simulink model "PruebaLEDs"  (R2023b)
settings: Solver=FixedStepAuto  StartTime=0.0  StopTime=inf  RelTol=1e-3
libraries: arduinolib x3
settings Model: Creator=Usuario_UMA  LastModifiedBy=Diego
settings OptimizationCC: DefaultParameterBehavior=Inlined  EnhancedBackFolding=on  PassReuseOutputArgsAs=Individual arguments  ZeroExternalMemoryAtStartup=off  ZeroInternalMemoryAtStartup=off  MaxStackSize=64  OptimizeBlockOrder=speed  DifferentSizesBufferReuse=on  OptimizationCustomize=off  EfficientTunableParamExpr=on
settings DebuggingCC: ParameterTunabilityLossMsg=error
settings HardwareCC: ProdBitPerInt=16  ProdBitPerPointer=16  ProdBitPerSizeT=16  ProdBitPerPtrDiffT=16  ProdLargestAtomicFloat=None  ProdWordSize=8  ProdHWDeviceType=Atmel->AVR
settings SFSimCC: MATLABDynamicMemAlloc=off
settings RTWCC: Description=Embedded Coder  SystemTargetFile=ert.tlc  TemplateMakefile=ert_default_tmf  Toolchain=Arduino AVR  BuildConfiguration=Faster Runs
settings CodeAppCC: ForceParamTrailComments=on  IgnoreCustomStorageClasses=off  OperatorAnnotations=on  SimulinkDataObjDesc=on  SFDataObjDesc=on  InsertBlockDesc=on
settings ERTTargetCC: SupportContinuousTime=on  ExtModeTransport=3  ExtModeStaticAlloc=on  ExtModeStaticAllocSize=2048  ExtModeMexFile=ext_xcp  ExtModeIntrfLevel=Level2 - Open  ERTCustomFileTemplate=example_file_process.tlc

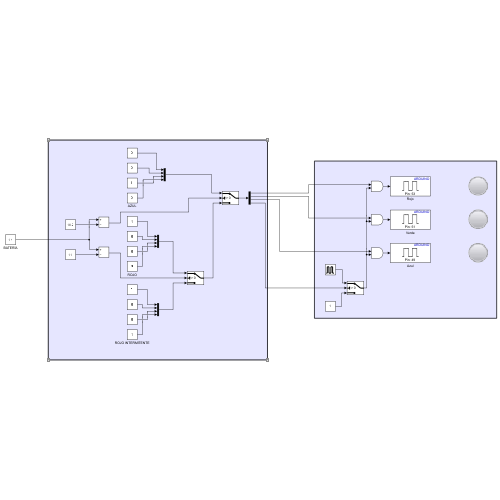
[thumbnail: Simulink's stored preview of the top-level diagram]
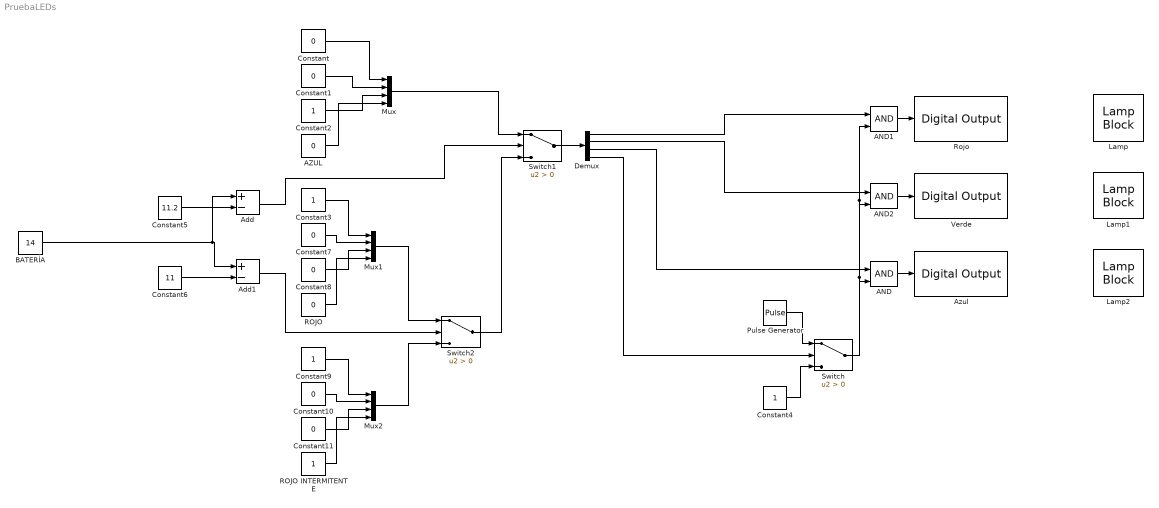
== system PruebaLEDs ==
  AND : Logic  IconShape=distinctive  AllPortsSameDT=off  OutDataTypeStr=boolean
  AND1 : Logic  IconShape=distinctive  AllPortsSameDT=off  OutDataTypeStr=boolean
  AND2 : Logic  IconShape=distinctive  AllPortsSameDT=off  OutDataTypeStr=boolean
  AZUL : Constant  Value=0
  Add : Sum  Inputs=+-
  Add1 : Sum  Inputs=+-
  Azul : arduinolib/Digital Output  pinNumber=49  Direction=output  blockPlatform=arduino
  BATERÍA : Constant  Value=14
  Constant{,1,7..8,10..11} (6 alike) : Constant  Value=0
  Constant{2..4,9} (4 alike) : Constant
  Constant5 : Constant  Value=11.2
  Constant6 : Constant  Value=11
  Demux : Demux
  Lamp : LampBlock  LabelPosition=Hide
  Lamp1 : LampBlock  LabelPosition=Hide
  Lamp2 : LampBlock  LabelPosition=Hide
  Mux : Mux
  Mux1 : Mux
  Mux2 : Mux
  Pulse Generator : DiscretePulseGenerator  PulseType=Time based  Period=1  PulseWidth=50
  ROJO : Constant  Value=0
  ROJO INTERMITENTE : Constant
  Rojo : arduinolib/Digital Output  pinNumber=53  Direction=output  blockPlatform=arduino
  Switch : Switch  Criteria=u2 > Threshold  SaturateOnIntegerOverflow=off  InputSameDT=off
  Switch1 : Switch  Criteria=u2 > Threshold  SaturateOnIntegerOverflow=off  InputSameDT=off
  Switch2 : Switch  Criteria=u2 > Threshold  SaturateOnIntegerOverflow=off  InputSameDT=off
  Verde : arduinolib/Digital Output  pinNumber=51  Direction=output  blockPlatform=arduino
  wires:
  AND/1 -> Azul/1
  Switch/1 -> AND2/2, AND1/2, AND/2
  Pulse Generator/1 -> Switch/1
  Constant4/1 -> Switch/3
  AND1/1 -> Rojo/1
  AND2/1 -> Verde/1
  Constant/1 -> Mux/1
  Constant1/1 -> Mux/2
  Constant2/1 -> Mux/3
  AZUL/1 -> Mux/4
  Constant3/1 -> Mux1/1
  Constant7/1 -> Mux1/2
  Constant8/1 -> Mux1/3
  ROJO/1 -> Mux1/4
  Constant9/1 -> Mux2/1
  Constant10/1 -> Mux2/2
  Constant11/1 -> Mux2/3
  ROJO INTERMITENTE/1 -> Mux2/4
  BATERÍA/1 -> Add/1, Add1/1
  Constant5/1 -> Add/2
  Constant6/1 -> Add1/2
  Add/1 -> Switch1/2
  Mux/1 -> Switch1/1
  Mux1/1 -> Switch2/1
  Add1/1 -> Switch2/2
  Mux2/1 -> Switch2/3
  Switch2/1 -> Switch1/3
  Switch1/1 -> Demux/1
  Demux/1 -> AND1/1
  Demux/2 -> AND2/1
  Demux/3 -> AND/1
  Demux/4 -> Switch/2
